simulink model "Md30StEnCtrl"  (R2018b)
settings: Solver=FixedStepDiscrete  StartTime=0.0  StopTime=10.0  FixedStep=0.01  RelTol=1e-3
undefined symbols (not defined in the file or in its folder): data, KeSMSuFirstRwStFwdBkwdPosDelta_Val, KeSMSw4SSecRwRtStLgrstOtwdInwdClosePos1_Val, KeSMSw4SSecRwRtStLgrstUpwdDnwdClosePos1_Val, KeSMSw4SSecRwRtStLgrstUpwdDnwdClosePos2_Val, KeSMSw4SSecRwRtStLgrstUpwdDnwdOpenPos1_Val, PassStBkReclnEn_Clear, PassStBkReclnEn_Set, PassStCshnFldEn_Clear, PassStCshnFldEn_Set, PassStFwdBkwdEn_Clear, PassStFwdBkwdEn_Set, SecRwRtStLgrstInwdOtwdEn_Clear, SecRwRtStLgrstInwdOtwdEn_Set, SecRwRtStLgrstUpwdDnwdEn_Clear, SecRwRtStLgrstUpwdDnwdEn_Set
libraries: simulink x3
settings Model: Creator=sn2xws  LastModifiedBy=sn55gm
settings Model: ModifiedHistory=|
  | 2024.6.27 V1.0.0 557模式流程V1.6
  | 2024.8.16 V3.0.0 增加firstTrig接口
  | 2024.8.19 V3.0.1前后位置判断时的减法加上括号保证运算顺序
  | 2024.11.6 V3.0.2模式流程V2.6 第一阶段增加收靠背动作
  | 2024.12.27 V3.0.3 BUG 965807 第一次靠背在位置判断应留余量
  | 25.07.15  V4.0.1 修改stage2前置条件
  | 25.7.31 V4.0.2 CR1100249
  | 25.8.11 V4.0.3 第一次完成后靠背到位置判断为alldone
  | 2025.09.03 V4.0.4 前后，折叠电机失败后退出
settings DataIOCC: SaveFormat=StructureWithTime
settings OptimizationCC: DefaultParameterBehavior=Inlined  EnhancedBackFolding=on  PassReuseOutputArgsAs=Individual arguments  ZeroExternalMemoryAtStartup=off  ZeroInternalMemoryAtStartup=off  OptimizeBlockOrder=speed  DifferentSizesBufferReuse=on  OptimizationCustomize=off
settings DebuggingCC: ParameterTunabilityLossMsg=error
settings SFSimCC: MATLABDynamicMemAlloc=off
settings RTWCC: SystemTargetFile=autosar.tlc  GenCodeOnly=on  TemplateMakefile=ert_default_tmf  Description=AUTOSAR  GenerateReport=on  IncludeHyperlinkInReport=on  LaunchReport=on  GenerateTraceInfo=on  GenerateTraceReport=on  GenerateTraceReportSl=on  GenerateTraceReportSf=on  GenerateTraceReportEml=on
settings CodeAppCC: ForceParamTrailComments=on  IgnoreCustomStorageClasses=off  OperatorAnnotations=on  SimulinkDataObjDesc=on  SFDataObjDesc=on  InsertBlockDesc=on
settings STFCustomTargetCC: TargetLangStandard=C99 (ISO)  MultiwordLength=256  ParMdlRefBuildCompliant=on  CompOptLevelCompliant=on  IncludeMdlTerminateFcn=off  CombineOutputUpdateFcns=on  SuppressErrorStatus=on  ERTCustomFileBanners=on  SupportNonFinite=off  SupportComplex=off  SupportContinuousTime=off  SupportNonInlinedSFcns=off  RemoveResetFunc=on  MATLABClassNameForMDSCustomization=Simulink.SoftwareTarget.ERTCustomization  AutosarCompliant=on  UseToolchainInfoCompliant=on  LookupTableObjectStructAxisOrder=2,1,3,4,...  LUTObjectStructOrderEvenSpacing=Size,Table,Breakpoints  SystemTargetFile=autosar.tlc
settings ERTTargetCC: TargetLangStandard=C99 (ISO)  ConcurrentExecutionCompliant=off  IncludeMdlTerminateFcn=off  SuppressErrorStatus=on  SupportNonFinite=off  SupportComplex=off  ModelStepFunctionPrototypeControlCompliant=off  CPPClassGenCompliant=off  AutosarCompliant=on  LookupTableObjectStructAxisOrder=2,1,3,4,...  LUTObjectStructOrderEvenSpacing=Size,Table,Breakpoints  InlinedParameterPlacement=NonHierarchical  ERTCustomFileTemplate=example_file_process.tlc  ERTFilePackagingFormat=Compact

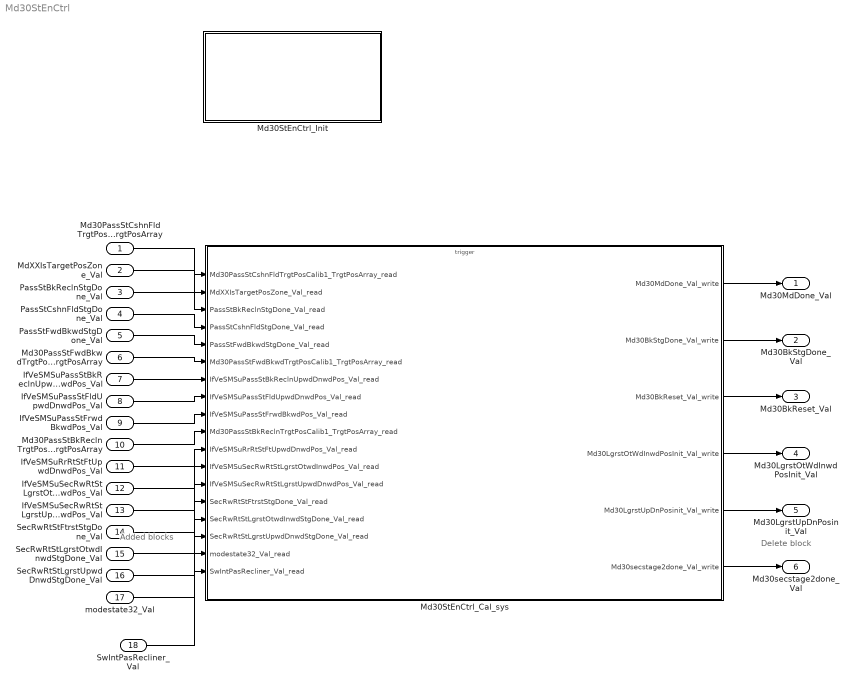
== system Md30StEnCtrl ==
  note: Delete block
  note: Added blocks
  Md30PassStCshnFldTrgtPosCalib1_TrgtPosArray : Inport  Description=|  OutDataTypeStr=uint16  PortDimensions=3
      | 0:Pos
      | 1:Max
      | 2:Min
  MdXXIsTargetPosZone_Val : Inport  Port=2  OutDataTypeStr=uint32  PortDimensions=1
  PassStBkReclnStgDone_Val : Inport  Port=3  OutDataTypeStr=boolean  PortDimensions=1
  PassStCshnFldStgDone_Val : Inport  Port=4  OutDataTypeStr=boolean  PortDimensions=1
  PassStFwdBkwdStgDone_Val : Inport  Port=5  OutDataTypeStr=boolean  PortDimensions=1
  Md30PassStFwdBkwdTrgtPosCalib1_TrgtPosArray : Inport  Description=|  Port=6  OutDataTypeStr=uint16  PortDimensions=3
      | 0:Pos
      | 1:Max
      | 2:Min
  IfVeSMSuPassStBkReclnUpwdDnwdPos_Val : Inport  Port=7  OutDataTypeStr=uint16  PortDimensions=1
  IfVeSMSuPassStFldUpwdDnwdPos_Val : Inport  Port=8  OutDataTypeStr=uint16  PortDimensions=1
  IfVeSMSuPassStFrwdBkwdPos_Val : Inport  Port=9  OutDataTypeStr=uint16  PortDimensions=1
  Md30PassStBkReclnTrgtPosCalib1_TrgtPosArray : Inport  Description=|  Port=10  OutDataTypeStr=uint16  PortDimensions=3
      | 0:Pos
      | 1:Max
      | 2:Min
  IfVeSMSuRrRtStFtUpwdDnwdPos_Val : Inport  Port=11  OutDataTypeStr=uint16  PortDimensions=1
  IfVeSMSuSecRwRtStLgrstOtwdInwdPos_Val : Inport  Port=12  OutDataTypeStr=uint16  PortDimensions=1
  IfVeSMSuSecRwRtStLgrstUpwdDnwdPos_Val : Inport  Port=13  OutDataTypeStr=uint16  PortDimensions=1
  SecRwRtStFtrstStgDone_Val : Inport  Port=14  OutDataTypeStr=boolean  PortDimensions=1
  SecRwRtStLgrstOtwdInwdStgDone_Val : Inport  Port=15  OutDataTypeStr=boolean  PortDimensions=1
  SecRwRtStLgrstUpwdDnwdStgDone_Val : Inport  Port=16  OutDataTypeStr=boolean  PortDimensions=1
  modestate32_Val : Inport  Port=17  OutDataTypeStr=uint32  PortDimensions=1
  SwIntPasRecliner_Val : Inport  Port=18  OutDataTypeStr=boolean  PortDimensions=1
  Md30StEnCtrl_Cal_sys : Subsystem
  Md30StEnCtrl_Init : Subsystem
  Md30MdDone_Val : Outport  OutDataTypeStr=uint8  PortDimensions=1
  Md30BkStgDone_Val : Outport  Port=2  OutDataTypeStr=boolean  PortDimensions=1
  Md30BkReset_Val : Outport  Port=3  OutDataTypeStr=boolean  PortDimensions=1
  Md30LgrstOtWdInwdPosInit_Val : Outport  Port=4  OutDataTypeStr=uint16  PortDimensions=1
  Md30LgrstUpDnPosinit_Val : Outport  Port=5  OutDataTypeStr=uint16  PortDimensions=1
  Md30secstage2done_Val : Outport  Port=6  OutDataTypeStr=boolean  PortDimensions=1
  wires:
  Md30PassStCshnFldTrgtPosCalib1_TrgtPosArray/1 -> Md30StEnCtrl_Cal_sys/1(Md30PassStCshnFldTrgtPosCalib1_TrgtPosArray_read)
  MdXXIsTargetPosZone_Val/1 -> Md30StEnCtrl_Cal_sys/2(MdXXIsTargetPosZone_Val_read)
  PassStBkReclnStgDone_Val/1 -> Md30StEnCtrl_Cal_sys/3(PassStBkReclnStgDone_Val_read)
  PassStCshnFldStgDone_Val/1 -> Md30StEnCtrl_Cal_sys/4(PassStCshnFldStgDone_Val_read)
  PassStFwdBkwdStgDone_Val/1 -> Md30StEnCtrl_Cal_sys/5(PassStFwdBkwdStgDone_Val_read)
  Md30StEnCtrl_Cal_sys/1(Md30MdDone_Val_write) -> Md30MdDone_Val/1
  Md30StEnCtrl_Cal_sys/2(Md30BkStgDone_Val_write) -> Md30BkStgDone_Val/1
  Md30PassStFwdBkwdTrgtPosCalib1_TrgtPosArray/1 -> Md30StEnCtrl_Cal_sys/6(Md30PassStFwdBkwdTrgtPosCalib1_TrgtPosArray_read)
  IfVeSMSuPassStBkReclnUpwdDnwdPos_Val/1 -> Md30StEnCtrl_Cal_sys/7(IfVeSMSuPassStBkReclnUpwdDnwdPos_Val_read)
  IfVeSMSuPassStFldUpwdDnwdPos_Val/1 -> Md30StEnCtrl_Cal_sys/8(IfVeSMSuPassStFldUpwdDnwdPos_Val_read)
  IfVeSMSuPassStFrwdBkwdPos_Val/1 -> Md30StEnCtrl_Cal_sys/9(IfVeSMSuPassStFrwdBkwdPos_Val_read)
  Md30PassStBkReclnTrgtPosCalib1_TrgtPosArray/1 -> Md30StEnCtrl_Cal_sys/10(Md30PassStBkReclnTrgtPosCalib1_TrgtPosArray_read)
  Md30StEnCtrl_Cal_sys/3(Md30BkReset_Val_write) -> Md30BkReset_Val/1
  IfVeSMSuRrRtStFtUpwdDnwdPos_Val/1 -> Md30StEnCtrl_Cal_sys/11(IfVeSMSuRrRtStFtUpwdDnwdPos_Val_read)
  IfVeSMSuSecRwRtStLgrstOtwdInwdPos_Val/1 -> Md30StEnCtrl_Cal_sys/12(IfVeSMSuSecRwRtStLgrstOtwdInwdPos_Val_read)
  IfVeSMSuSecRwRtStLgrstUpwdDnwdPos_Val/1 -> Md30StEnCtrl_Cal_sys/13(IfVeSMSuSecRwRtStLgrstUpwdDnwdPos_Val_read)
  SecRwRtStFtrstStgDone_Val/1 -> Md30StEnCtrl_Cal_sys/14(SecRwRtStFtrstStgDone_Val_read)
  SecRwRtStLgrstOtwdInwdStgDone_Val/1 -> Md30StEnCtrl_Cal_sys/15(SecRwRtStLgrstOtwdInwdStgDone_Val_read)
  SecRwRtStLgrstUpwdDnwdStgDone_Val/1 -> Md30StEnCtrl_Cal_sys/16(SecRwRtStLgrstUpwdDnwdStgDone_Val_read)
  modestate32_Val/1 -> Md30StEnCtrl_Cal_sys/17(modestate32_Val_read)
  Md30StEnCtrl_Cal_sys/4(Md30LgrstOtWdInwdPosInit_Val_write) -> Md30LgrstOtWdInwdPosInit_Val/1
  Md30StEnCtrl_Cal_sys/5(Md30LgrstUpDnPosinit_Val_write) -> Md30LgrstUpDnPosinit_Val/1
  Md30StEnCtrl_Cal_sys/6(Md30secstage2done_Val_write) -> Md30secstage2done_Val/1
  SwIntPasRecliner_Val/1 -> Md30StEnCtrl_Cal_sys/18(SwIntPasRecliner_Val_read)

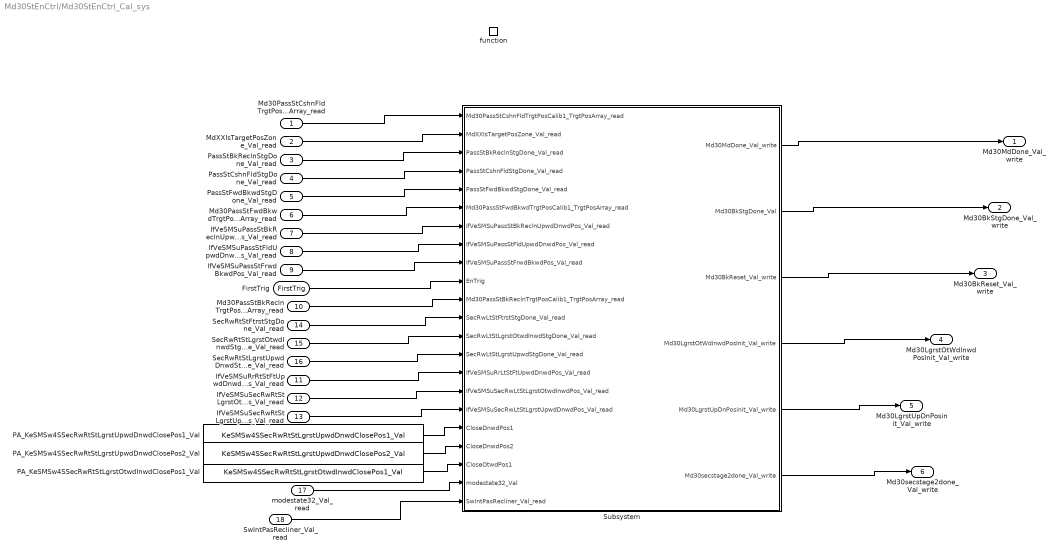
== system Md30StEnCtrl/Md30StEnCtrl_Cal_sys ==
  Md30PassStCshnFldTrgtPosCalib1_TrgtPosArray_read : Inport
  MdXXIsTargetPosZone_Val_read : Inport  Port=2
  PassStBkReclnStgDone_Val_read : Inport  Port=3
  PassStCshnFldStgDone_Val_read : Inport  Port=4
  PassStFwdBkwdStgDone_Val_read : Inport  Port=5
  Md30PassStFwdBkwdTrgtPosCalib1_TrgtPosArray_read : Inport  Port=6
  IfVeSMSuPassStBkReclnUpwdDnwdPos_Val_read : Inport  Port=7
  IfVeSMSuPassStFldUpwdDnwdPos_Val_read : Inport  Port=8
  IfVeSMSuPassStFrwdBkwdPos_Val_read : Inport  Port=9
  Md30PassStBkReclnTrgtPosCalib1_TrgtPosArray_read : Inport  Port=10
  IfVeSMSuRrRtStFtUpwdDnwdPos_Val_read : Inport  Port=11
  IfVeSMSuSecRwRtStLgrstOtwdInwdPos_Val_read : Inport  Port=12
  IfVeSMSuSecRwRtStLgrstUpwdDnwdPos_Val_read : Inport  Port=13
  SecRwRtStFtrstStgDone_Val_read : Inport  Port=14
  SecRwRtStLgrstOtwdInwdStgDone_Val_read : Inport  Port=15
  SecRwRtStLgrstUpwdDnwdStgDone_Val_read : Inport  Port=16
  modestate32_Val_read : Inport  Port=17
  SwIntPasRecliner_Val_read : Inport  Port=18
  function : TriggerPort  TriggerType=function-call  IsSimulinkFunction=on  FunctionName=Md30StEnCtrl_Cal  VariantControl=(inherit)
  PA_KeSMSw4SSecRwRtStLgrstOtwdInwdClosePos1_Val : Constant  Value=KeSMSw4SSecRwRtStLgrstOtwdInwdClosePos1_Val
  PA_KeSMSw4SSecRwRtStLgrstUpwdDnwdClosePos1_Val : Constant  Value=KeSMSw4SSecRwRtStLgrstUpwdDnwdClosePos1_Val
  PA_KeSMSw4SSecRwRtStLgrstUpwdDnwdClosePos2_Val : Constant  Value=KeSMSw4SSecRwRtStLgrstUpwdDnwdClosePos2_Val
  Subsystem : Subsystem
  FirstTrig : ArgIn  OutDataTypeStr=boolean  ArgumentName=FirstTrig
  Md30MdDone_Val_write : Outport
      settings: EnsureOutportIsVirtual=on
  Md30BkStgDone_Val_write : Outport  Port=2
      settings: EnsureOutportIsVirtual=on
  Md30BkReset_Val_write : Outport  Port=3
      settings: EnsureOutportIsVirtual=on
  Md30LgrstOtWdInwdPosInit_Val_write : Outport  Port=4
      settings: EnsureOutportIsVirtual=on
  Md30LgrstUpDnPosinit_Val_write : Outport  Port=5
      settings: EnsureOutportIsVirtual=on
  Md30secstage2done_Val_write : Outport  Port=6
      settings: EnsureOutportIsVirtual=on
  wires:
  Md30PassStCshnFldTrgtPosCalib1_TrgtPosArray_read/1 -> Subsystem/1(Md30PassStCshnFldTrgtPosCalib1_TrgtPosArray_read)
  MdXXIsTargetPosZone_Val_read/1 -> Subsystem/2(MdXXIsTargetPosZone_Val_read)
  PassStBkReclnStgDone_Val_read/1 -> Subsystem/3(PassStBkReclnStgDone_Val_read)
  PassStCshnFldStgDone_Val_read/1 -> Subsystem/4(PassStCshnFldStgDone_Val_read)
  PassStFwdBkwdStgDone_Val_read/1 -> Subsystem/5(PassStFwdBkwdStgDone_Val_read)
  Subsystem/1(Md30MdDone_Val_write) -> Md30MdDone_Val_write/1
  Subsystem/2(Md30BkStgDone_Val) -> Md30BkStgDone_Val_write/1
  Md30PassStFwdBkwdTrgtPosCalib1_TrgtPosArray_read/1 -> Subsystem/6(Md30PassStFwdBkwdTrgtPosCalib1_TrgtPosArray_read)
  IfVeSMSuPassStBkReclnUpwdDnwdPos_Val_read/1 -> Subsystem/7(IfVeSMSuPassStBkReclnUpwdDnwdPos_Val_read)
  IfVeSMSuPassStFldUpwdDnwdPos_Val_read/1 -> Subsystem/8(IfVeSMSuPassStFldUpwdDnwdPos_Val_read)
  IfVeSMSuPassStFrwdBkwdPos_Val_read/1 -> Subsystem/9(IfVeSMSuPassStFrwdBkwdPos_Val_read)
  Md30PassStBkReclnTrgtPosCalib1_TrgtPosArray_read/1 -> Subsystem/11(Md30PassStBkReclnTrgtPosCalib1_TrgtPosArray_read)
  FirstTrig/1 -> Subsystem/10(EnTrig)
  Subsystem/3(Md30BkReset_Val_write) -> Md30BkReset_Val_write/1
  IfVeSMSuRrRtStFtUpwdDnwdPos_Val_read/1 -> Subsystem/15(IfVeSMSuRrLtStFtUpwdDnwdPos_Val_read)
  IfVeSMSuSecRwRtStLgrstUpwdDnwdPos_Val_read/1 -> Subsystem/17(IfVeSMSuSecRwLtStLgrstUpwdDnwdPos_Val_read)
  SecRwRtStLgrstOtwdInwdStgDone_Val_read/1 -> Subsystem/13(SecRwLtStLgrstOtwdInwdStgDone_Val_read)
  SecRwRtStFtrstStgDone_Val_read/1 -> Subsystem/12(SecRwLtStFtrstStgDone_Val_read)
  SecRwRtStLgrstUpwdDnwdStgDone_Val_read/1 -> Subsystem/14(SecRwLtStLgrstUpwdStgDone_Val_read)
  IfVeSMSuSecRwRtStLgrstOtwdInwdPos_Val_read/1 -> Subsystem/16(IfVeSMSuSecRwLtStLgrstOtwdInwdPos_Val_read)
  PA_KeSMSw4SSecRwRtStLgrstUpwdDnwdClosePos1_Val/1 -> Subsystem/18(CloseDnwdPos1)
  PA_KeSMSw4SSecRwRtStLgrstOtwdInwdClosePos1_Val/1 -> Subsystem/20(CloseOtwdPos1)
  PA_KeSMSw4SSecRwRtStLgrstUpwdDnwdClosePos2_Val/1 -> Subsystem/19(CloseDnwdPos2)
  modestate32_Val_read/1 -> Subsystem/21(modestate32_Val)
  Subsystem/4(Md30LgrstOtWdInwdPosInit_Val_write) -> Md30LgrstOtWdInwdPosInit_Val_write/1
  Subsystem/5(Md30LgrstUpDnPosinit_Val_write) -> Md30LgrstUpDnPosinit_Val_write/1
  Subsystem/6(Md30secstage2done_Val_write) -> Md30secstage2done_Val_write/1
  SwIntPasRecliner_Val_read/1 -> Subsystem/22(SwIntPasRecliner_Val_read)

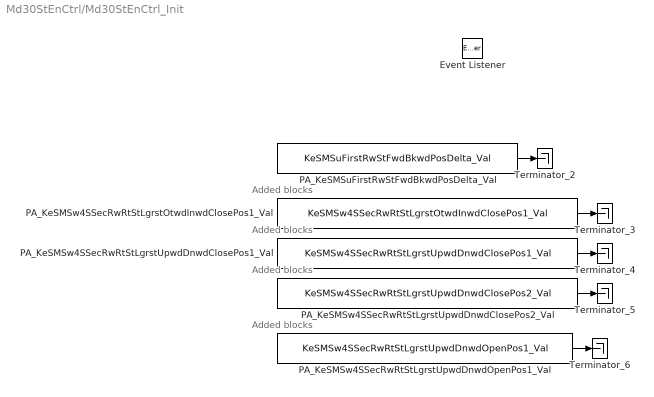
== system Md30StEnCtrl/Md30StEnCtrl_Init ==
  note: Added blocks
  note: Added blocks
  note: Added blocks
  note: Added blocks
  Event Listener : EventListener  EventName=reset
  PA_KeSMSuFirstRwStFwdBkwdPosDelta_Val : Constant  Value=KeSMSuFirstRwStFwdBkwdPosDelta_Val
  PA_KeSMSw4SSecRwRtStLgrstOtwdInwdClosePos1_Val : Constant  Value=KeSMSw4SSecRwRtStLgrstOtwdInwdClosePos1_Val
  PA_KeSMSw4SSecRwRtStLgrstUpwdDnwdClosePos1_Val : Constant  Value=KeSMSw4SSecRwRtStLgrstUpwdDnwdClosePos1_Val
  PA_KeSMSw4SSecRwRtStLgrstUpwdDnwdClosePos2_Val : Constant  Value=KeSMSw4SSecRwRtStLgrstUpwdDnwdClosePos2_Val
  PA_KeSMSw4SSecRwRtStLgrstUpwdDnwdOpenPos1_Val : Constant  Value=KeSMSw4SSecRwRtStLgrstUpwdDnwdOpenPos1_Val
  Terminator_{2..6} (5 alike) : Terminator
  wires:
  PA_KeSMSuFirstRwStFwdBkwdPosDelta_Val/1 -> Terminator_2/1
  PA_KeSMSw4SSecRwRtStLgrstOtwdInwdClosePos1_Val/1 -> Terminator_3/1
  PA_KeSMSw4SSecRwRtStLgrstUpwdDnwdClosePos1_Val/1 -> Terminator_4/1
  PA_KeSMSw4SSecRwRtStLgrstUpwdDnwdClosePos2_Val/1 -> Terminator_5/1
  PA_KeSMSw4SSecRwRtStLgrstUpwdDnwdOpenPos1_Val/1 -> Terminator_6/1

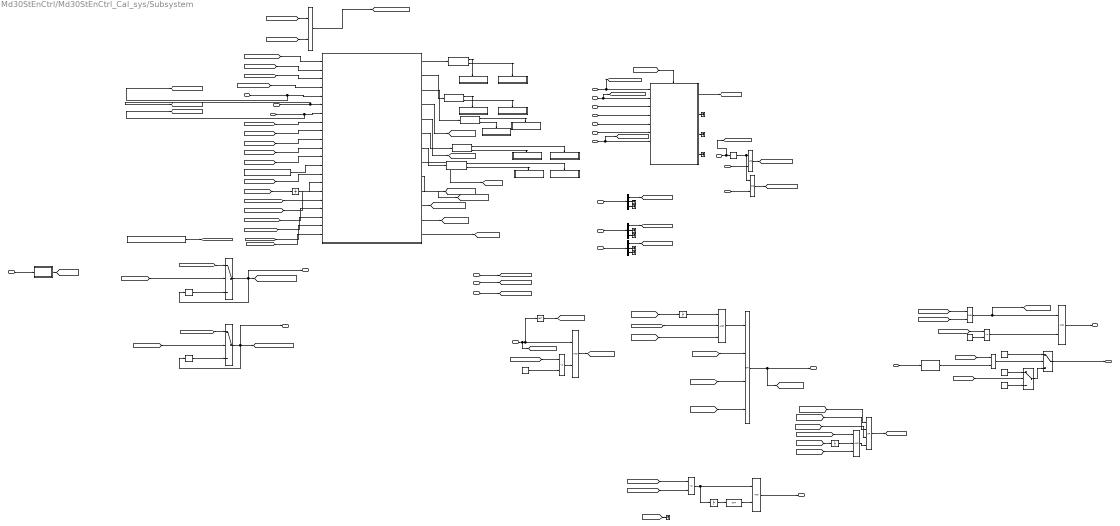
== system Md30StEnCtrl/Md30StEnCtrl_Cal_sys/Subsystem ==
  Md30PassStCshnFldTrgtPosCalib1_TrgtPosArray_read : Inport
  MdXXIsTargetPosZone_Val_read : Inport  Port=2
  PassStBkReclnStgDone_Val_read : Inport  Port=3
  PassStCshnFldStgDone_Val_read : Inport  Port=4
  PassStFwdBkwdStgDone_Val_read : Inport  Port=5
  Md30PassStFwdBkwdTrgtPosCalib1_TrgtPosArray_read : Inport  Port=6
  IfVeSMSuPassStBkReclnUpwdDnwdPos_Val_read : Inport  Port=7
  IfVeSMSuPassStFldUpwdDnwdPos_Val_read : Inport  Port=8
  IfVeSMSuPassStFrwdBkwdPos_Val_read : Inport  Port=9
  EnTrig : Inport  Port=10
  Md30PassStBkReclnTrgtPosCalib1_TrgtPosArray_read : Inport  Port=11
  SecRwLtStFtrstStgDone_Val_read : Inport  Port=12
  SecRwLtStLgrstOtwdInwdStgDone_Val_read : Inport  Port=13
  SecRwLtStLgrstUpwdStgDone_Val_read : Inport  Port=14
  IfVeSMSuRrLtStFtUpwdDnwdPos_Val_read : Inport  Port=15
  IfVeSMSuSecRwLtStLgrstOtwdInwdPos_Val_read : Inport  Port=16
  IfVeSMSuSecRwLtStLgrstUpwdDnwdPos_Val_read : Inport  Port=17
  CloseDnwdPos1 : Inport  Port=18
  CloseDnwdPos2 : Inport  Port=19
  CloseOtwdPos1 : Inport  Port=20
  modestate32_Val : Inport  Port=21
  SwIntPasRecliner_Val_read : Inport  Port=22
  32BitSelector : Subsystem  mask(32 Bit Selector){BitNum=29}
      mask prompts: BitNum "Select Bit Number"
      mask help: Allows selection of a particular bit (0-31) out of a packed word up to 32 bits long. Output will be true if the bit number selected via the mask parameter is equal to one.
      mask TypeOptions BitNum: 0 | 1 | 2 | 3 | 4 | 5 | 6 | 7 | 8 | 9 | 10 | 11 | 12 | 13 | 14 | 15 | 16 | 17 | 18 | 19 | 20 | 21 | 22 | 23 | 24 | 25 | 26 | 27 | 28 | 29 | 30 | 31
      mask Display:
      | text(0.5, 0.8,'BIT','horizontalAlignment','center')
      | text(0.5, 0.5,'SELECTOR','horizontalAlignment','center')
      | text(0.5, 0.2,['-- Bit ',char(get_param(gcb,'BitNum')),' --'],'horizontalAlignment','center')
  32BitSelector1 : Subsystem  mask(32 Bit Selector){BitNum=29}
      mask prompts: BitNum "Select Bit Number"
      mask help: Allows selection of a particular bit (0-31) out of a packed word up to 32 bits long. Output will be true if the bit number selected via the mask parameter is equal to one.
      mask TypeOptions BitNum: 0 | 1 | 2 | 3 | 4 | 5 | 6 | 7 | 8 | 9 | 10 | 11 | 12 | 13 | 14 | 15 | 16 | 17 | 18 | 19 | 20 | 21 | 22 | 23 | 24 | 25 | 26 | 27 | 28 | 29 | 30 | 31
      mask Display:
      | text(0.5, 0.8,'BIT','horizontalAlignment','center')
      | text(0.5, 0.5,'SELECTOR','horizontalAlignment','center')
      | text(0.5, 0.2,['-- Bit ',char(get_param(gcb,'BitNum')),' --'],'horizontalAlignment','center')
  Chart : Stateflow chart  TreatAsAtomicUnit=on
  Compare To Constant : simulink/Logic and Bit Operations/Compare To Constant  relop===  const=1  OutDataTypeStr=boolean
  Constant : Constant  Value=40  OutDataTypeStr=uint16
  Constant1 : Constant  OutDataTypeStr=uint8
  Constant2 : Constant  Value=2  OutDataTypeStr=uint8
  Constant3 : Constant  Value=0  OutDataTypeStr=uint8
  Constant4 : Constant  Value=120  OutDataTypeStr=uint16
  Delay1 : Delay  DelayLength=1
  Delay3 : Delay  DelayLength=1
  Demux : Demux  Outputs=3
  Demux1 : Demux  Outputs=3
  Demux2 : Demux  Outputs=3
  If Action Subsystem1 : Subsystem  TreatAsAtomicUnit=on
  If Action Subsystem11 : Subsystem  TreatAsAtomicUnit=on
  If Action Subsystem14 : Subsystem  TreatAsAtomicUnit=on
  If Action Subsystem2 : Subsystem  TreatAsAtomicUnit=on
  If Action Subsystem3 : Subsystem  TreatAsAtomicUnit=on
  If Action Subsystem4 : Subsystem  TreatAsAtomicUnit=on
  If Action Subsystem5 : Subsystem  TreatAsAtomicUnit=on
  If Action Subsystem6 : Subsystem  TreatAsAtomicUnit=on
  If Action Subsystem7 : Subsystem  TreatAsAtomicUnit=on
  If Action Subsystem8 : Subsystem  TreatAsAtomicUnit=on
  If{1..4,8} (5 alike) : If  IfExpression=u1
  Logical Operator{,3,5,9,13,24} (6 alike) : Logic  AllPortsSameDT=off  OutDataTypeStr=boolean
  Logical Operator1 : Logic  Inputs=3  AllPortsSameDT=off  OutDataTypeStr=boolean
  Logical Operator10 : Logic  Operator=OR  AllPortsSameDT=off  OutDataTypeStr=boolean
  Logical Operator2 : Logic  Operator=OR  Inputs=4  AllPortsSameDT=off  OutDataTypeStr=boolean
  Logical Operator22 : Logic  Inputs=3  AllPortsSameDT=off  OutDataTypeStr=boolean
  Logical Operator4 : Logic  Operator=NOT  AllPortsSameDT=off  OutDataTypeStr=boolean
  Logical Operator6 : Logic  Operator=NOT  AllPortsSameDT=off  OutDataTypeStr=boolean
  Logical Operator7 : Logic  Operator=OR  Inputs=4  AllPortsSameDT=off  OutDataTypeStr=boolean
  Logical Operator8 : Logic  Operator=OR  AllPortsSameDT=off  OutDataTypeStr=boolean
  PA_KeSMSuFirstRwStFwdBkwdPosDelta_Val : Constant  Value=KeSMSuFirstRwStFwdBkwdPosDelta_Val
  PA_KeSMSw4SSecRwRtStLgrstUpwdDnwdClosePos1_Val : Constant  Value=KeSMSw4SSecRwRtStLgrstUpwdDnwdOpenPos1_Val
  Relational Operator : RelationalOperator  Operator=<=  OutDataTypeStr=boolean  RndMeth=Simplest
  Relational Operator1 : RelationalOperator  Operator=<=  OutDataTypeStr=boolean  RndMeth=Simplest
  Relational Operator2 : RelationalOperator  Operator=<=  OutDataTypeStr=boolean  RndMeth=Simplest
  Subsystem : Subsystem
  Switch{,1..3} (4 alike) : Switch  Criteria=u2 > Threshold
  Terminator_{1..2,4..5,7..12} (10 alike) : Terminator
  Unit Delay{,1..3} (4 alike) : UnitDelay  SampleTime=-1
  Md30MdDone_Val_write : Outport
      settings: EnsureOutportIsVirtual=on
  Md30BkStgDone_Val : Outport  Port=2
      settings: EnsureOutportIsVirtual=on
  Md30BkReset_Val_write : Outport  Port=3
      settings: EnsureOutportIsVirtual=on
  Md30LgrstOtWdInwdPosInit_Val_write : Outport  Port=4
  Md30LgrstUpDnPosinit_Val_write : Outport  Port=5
  Md30secstage2done_Val_write : Outport  Port=6
  wires:
  Switch/1 -> Md30MdDone_Val_write/1
  PassStBkReclnStgDone_Val_read/1 -> [PassStBkReclnStgDone], Chart/5(PassStBkReclnStgDone)
  PassStCshnFldStgDone_Val_read/1 -> Chart/6(PassStCshnFldStgDone), [PassStCshnFldStgDone]
  PassStFwdBkwdStgDone_Val_read/1 -> Chart/7(PassStFwdBkwdStgDone), [PassStFwdBkwdStgDone]
  [AllDone] -> Logical Operator9/1
  Constant1/1 -> Switch/1
  Constant2/1 -> Switch1/1
  Switch1/1 -> Switch/3
  Constant3/1 -> Switch1/3
  Logical Operator9/1 -> Switch/2
  MdXXIsTargetPosZone_Val_read/1 -> 32BitSelector/1(x)
  [AllDone] -> Switch1/2
  Md30PassStFwdBkwdTrgtPosCalib1_TrgtPosArray_read/1 -> Demux/1
  Demux/1 -> [PassStFwdBkwdTrgtPos1]
  Demux1/1 -> [PassStCshnFldTrgtPos1]
  Md30PassStCshnFldTrgtPosCalib1_TrgtPosArray_read/1 -> Demux1/1
  [PassStFwdBkwdTrgtPos1] -> Chart/8(PassStFwdBkwdTrgtPos1)
  [PassStCshnFldTrgtPos1] -> Chart/9(PassStCshnFldTrgtPos1)
  IfVeSMSuPassStFrwdBkwdPos_Val_read/1 -> [PassStFwdBkwdPos]
  IfVeSMSuPassStFldUpwdDnwdPos_Val_read/1 -> [PassStFldUpwdDnwdPos]
  [PassStFldUpwdDnwdPos] -> Chart/10(PassStFldUpwdDnwdPos)
  [PassStFwdBkwdPos] -> Chart/11(PassStFwdBkwdPos)
  IfVeSMSuPassStBkReclnUpwdDnwdPos_Val_read/1 -> [PassStBkReclnUpwdDnwdPos]
  [PassStBkReclnUpwdDnwdPos] -> Chart/12(PassStBkReclnUpwdDnwdPos)
  Logical Operator/1 -> Logical Operator13/1, [BkStgDone]
  [PassStCshnFldStgDone] -> Logical Operator/2
  [BkStgDone] -> Unit Delay/1
  Unit Delay/1 -> Logical Operator1/1
  [PassStFwdBkwdStgDone] -> Logical Operator1/2
  Chart/1(PassStBkReclnEn) -> If8/1
  If8/1 -> If Action Subsystem14/Action
  If8/2 -> If Action Subsystem11/Action
  If1/2 -> If Action Subsystem1/Action
  If1/1 -> If Action Subsystem2/Action
  Chart/2(PassStCshnFldEn) -> If1/1
  If2/1 -> If Action Subsystem4/Action
  If2/2 -> If Action Subsystem3/Action
  Chart/3(PassStFwdBkwdEn) -> If2/1
  Demux/2 -> Terminator_4/1
  Demux/3 -> Terminator_5/1
  Demux1/2 -> Terminator_7/1
  Demux1/3 -> Terminator_8/1
  PA_KeSMSuFirstRwStFwdBkwdPosDelta_Val/1 -> Chart/13(KeSMSuFirstRwStFwdBkwdPosDelta)
  Chart/4(FwdBkwdFailflg) -> [FwdBkwdFailflg]
  Chart/5(CshnFldFailflg) -> [CshnFldFailflg]
  Logical Operator1/1 -> Logical Operator2/1
  [FwdBkwdFailflg] -> Logical Operator2/2
  [CshnFldFailflg] -> Logical Operator2/3
  [PassStBkReclnUpwdDnwdPos] -> Relational Operator/1
  Constant/1 -> Relational Operator/2
  [FirstBkDone] -> Logical Operator2/4
  Relational Operator/1 -> Logical Operator3/2
  Logical Operator3/1 -> [FirstBkDone]
  32BitSelector/1(y) -> Logical Operator9/2
  [PassStBkReclnStgDone] -> Logical Operator/1
  Demux2/3 -> Terminator_2/1
  Demux2/2 -> Terminator_1/1
  Demux2/1 -> [Md30PassStBkReclnTrgtPos1]
  Md30PassStBkReclnTrgtPosCalib1_TrgtPosArray_read/1 -> Demux2/1
  [Md30PassStBkReclnTrgtPos1] -> Chart/14(Md30PassStBkReclnTrgtPos1)
  [PassStFldUpwdDnwdPos] -> Relational Operator1/1
  [PassStCshnFldTrgtPos1] -> Relational Operator1/2
  Relational Operator1/1 -> Logical Operator5/1, Unit Delay1/1
  Unit Delay1/1 -> Logical Operator4/1
  Logical Operator4/1 -> Logical Operator5/2
  Logical Operator5/1 -> Md30BkReset_Val_write/1
  [NotFirstTime] -> Logical Operator1/3
  Logical Operator6/1 -> [NotFirstTime]
  SecRwLtStLgrstOtwdInwdStgDone_Val_read/1 -> Subsystem/7(In7), [SecRwLtStLgrstOtwdInwdStgDone]
  IfVeSMSuSecRwLtStLgrstUpwdDnwdPos_Val_read/1 -> [LgrstUpDnPos], Subsystem/1(In1)
  IfVeSMSuSecRwLtStLgrstOtwdInwdPos_Val_read/1 -> Subsystem/2(In2), [LgrstOtWdInwdPos]
  IfVeSMSuRrLtStFtUpwdDnwdPos_Val_read/1 -> Subsystem/3(In3)
  CloseDnwdPos1/1 -> Subsystem/4(In4)
  CloseDnwdPos2/1 -> Subsystem/5(In5)
  CloseOtwdPos1/1 -> Subsystem/6(In6)
  Subsystem/1(Out1) -> [failflg]
  Chart/13(TrigLgrstcls()) -> [TrigLgrstcls]
  [TrigLgrstcls] -> Subsystem/Trigger
  [stage2Done] -> Unit Delay3/1
  Relational Operator2/1 -> Logical Operator13/2
  [PassStBkReclnUpwdDnwdPos] -> Relational Operator2/1
  Constant4/1 -> Relational Operator2/2
  Logical Operator13/1 -> Md30BkStgDone_Val/1
  [SecRwLtStFtrstStgDone] -> Chart/4(SecRwLtStFtrstStgDone)
  [SecRwLtStLgrstUpwdStgDone] -> Chart/2(SecRwLtStLgrstUpwdStgDone)
  [SecRwLtStLgrstOtwdInwdStgDone] -> Chart/3(SecRwLtStLgrstOtwdInwdStgDone)
  modestate32_Val/1 -> 32BitSelector1/1(x)
  32BitSelector1/1(y) -> [Mode30]
  [EnTrig] -> Switch2/2
  [LgrstOtWdInwdPos] -> Switch2/1
  Delay1/1 -> Switch2/3
  Delay3/1 -> Switch3/3
  [LgrstUpDnPos] -> Switch3/1
  Switch2/1 -> Md30LgrstOtWdInwdPosInit_Val_write/1, Delay1/1, [LgrstOtWdInwdPosInit]
  [LgrstOtWdInwdPosInit] -> Chart/16(LgrstOtWdInwdPosInit)
  [LgrstUpDnPosinit] -> Chart/17(LgrstUpDnPosinit)
  [LgrstOtWdInwdPos] -> Chart/18(LgrstOtWdInwdPos)
  [LgrstUpDnPos] -> Chart/19(LgrstUpDnPos)
  Switch3/1 -> Delay3/1, Md30LgrstUpDnPosinit_Val_write/1, [LgrstUpDnPosinit]
  [LgrstUpwdDnwdOpenPos1] -> Chart/20(LgrstUpwdDnwdOpenPos1)
  Chart/6(SecRwLtStLgrstUpwdEn) -> If3/1
  Chart/8(LgrstUpwdfailflg) -> [LgrstUpwdfailflg]
  Chart/9(stage2LgrstUpwdStgDone) -> [stage2LgrstUpwdStgDone]
  Chart/10(stage2LgrstOtwdInwdStgDone) -> [stage2LgrstOtwdInwdStgDone]
  Logical Operator2/1 -> [stage2Done], Md30secstage2done_Val_write/1
  [stage2Done] -> Unit Delay2/1
  [LgrstUpwdfailflg] -> Terminator_9/1
  PA_KeSMSw4SSecRwRtStLgrstUpwdDnwdClosePos1_Val/1 -> [LgrstUpwdDnwdOpenPos1]
  [SecRwLtStLgrstOtwdInwdStgDone] -> Logical Operator24/2
  [SecRwLtStLgrstUpwdStgDone] -> Logical Operator24/1
  [stage1Done] -> Chart/1(stage1Done)
  If3/1 -> If Action Subsystem5/Action
  If4/2 -> If Action Subsystem8/Action
  If4/1 -> If Action Subsystem7/Action
  Chart/7(SecRwLtStLgrstOtwdInwdEn) -> If4/1
  Subsystem/2(Out2) -> Terminator_10/1
  Subsystem/3(Out3) -> Terminator_11/1
  Subsystem/4(Out4) -> Terminator_12/1
  Unit Delay3/1 -> Chart/15(stage2Done)
  EnTrig/1 -> [EnTrig], Logical Operator6/1, Logical Operator3/1
  [EnTrig] -> Switch3/2
  If3/2 -> If Action Subsystem6/Action
  [stage1Done] -> Logical Operator22/1
  Unit Delay2/1 -> Logical Operator22/2
  [NotFirstTime] -> Logical Operator22/3
  Chart/11(LgrstUpDnPosfail) -> [LgrstUpDnPosfail]
  Chart/12(LgrstOtWdInwdPosfail) -> [LgrstOtWdInwdPosfail]
  Logical Operator24/1 -> [stage1Done]
  Logical Operator22/1 -> Logical Operator7/4
  [FirstBkDone] -> Logical Operator7/3
  Logical Operator7/1 -> [AllDone]
  [FwdBkwdFailflg] -> Logical Operator7/2
  [CshnFldFailflg] -> Logical Operator7/1
  Compare To Constant/1 -> Logical Operator10/1, Logical Operator8/1
  SecRwLtStLgrstUpwdStgDone_Val_read/1 -> Logical Operator8/2
  Logical Operator8/1 -> [SecRwLtStLgrstUpwdStgDone]
  SecRwLtStFtrstStgDone_Val_read/1 -> Logical Operator10/2
  Logical Operator10/1 -> [SecRwLtStFtrstStgDone]
  SwIntPasRecliner_Val_read/1 -> [SwIntPasRecliner], Compare To Constant/1
  [SwIntPasRecliner] -> Chart/21(SwIntPasRecliner)

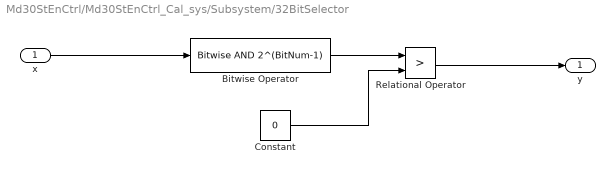
== system Md30StEnCtrl/Md30StEnCtrl_Cal_sys/Subsystem/32BitSelector ==
  x : Inport
  Bitwise Operator : simulink/Logic and Bit Operations/Bitwise Operator  logicop=AND  UseBitMask=on  BitMask=2^(BitNum-1)  BitMaskRealWorld=Stored Integer
  Constant : Constant  Value=0  OutDataTypeStr=uint32
  Relational Operator : RelationalOperator  Operator=>  OutDataTypeStr=boolean  RndMeth=Simplest
  y : Outport
  wires:
  Relational Operator/1 -> y/1
  Constant/1 -> Relational Operator/2
  x/1 -> Bitwise Operator/1
  Bitwise Operator/1 -> Relational Operator/1

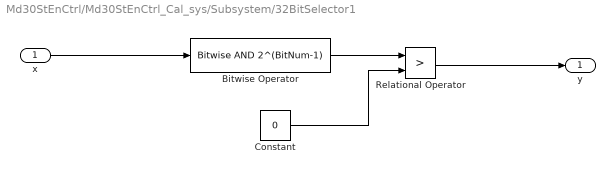
== system Md30StEnCtrl/Md30StEnCtrl_Cal_sys/Subsystem/32BitSelector1 ==
  x : Inport
  Bitwise Operator : simulink/Logic and Bit Operations/Bitwise Operator  logicop=AND  UseBitMask=on  BitMask=2^(BitNum-1)  BitMaskRealWorld=Stored Integer
  Constant : Constant  Value=0  OutDataTypeStr=uint32
  Relational Operator : RelationalOperator  Operator=>  OutDataTypeStr=boolean  RndMeth=Simplest
  y : Outport
  wires:
  Relational Operator/1 -> y/1
  Constant/1 -> Relational Operator/2
  x/1 -> Bitwise Operator/1
  Bitwise Operator/1 -> Relational Operator/1

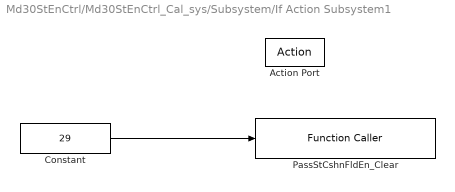
== system Md30StEnCtrl/Md30StEnCtrl_Cal_sys/Subsystem/If Action Subsystem1 ==
  Action Port : ActionPort  ActionType=else
  Constant : Constant  Value=29  OutDataTypeStr=uint8
  PassStCshnFldEn_Clear : FunctionCaller  FunctionPrototype=PassStCshnFldEn_Clear(data)  InputArgumentSpecifications=uint8(1)
  wires:
  Constant/1 -> PassStCshnFldEn_Clear/1

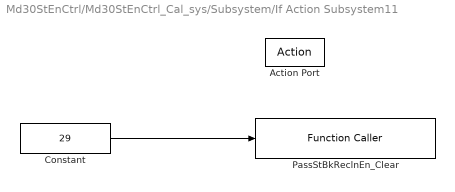
== system Md30StEnCtrl/Md30StEnCtrl_Cal_sys/Subsystem/If Action Subsystem11 ==
  Action Port : ActionPort  ActionType=else
  Constant : Constant  Value=29  OutDataTypeStr=uint8
  PassStBkReclnEn_Clear : FunctionCaller  FunctionPrototype=PassStBkReclnEn_Clear(data)  InputArgumentSpecifications=uint8(1)
  wires:
  Constant/1 -> PassStBkReclnEn_Clear/1

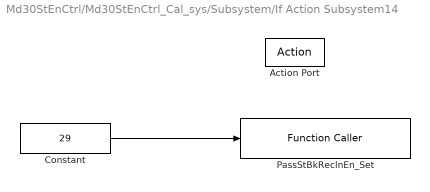
== system Md30StEnCtrl/Md30StEnCtrl_Cal_sys/Subsystem/If Action Subsystem14 ==
  Action Port : ActionPort  ActionType=then
  Constant : Constant  Value=29  OutDataTypeStr=uint8
  PassStBkReclnEn_Set : FunctionCaller  FunctionPrototype=PassStBkReclnEn_Set(data)  InputArgumentSpecifications=uint8(1)
  wires:
  Constant/1 -> PassStBkReclnEn_Set/1

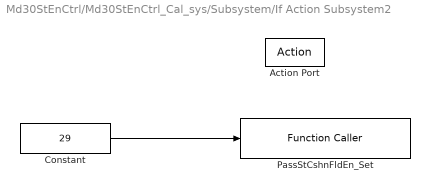
== system Md30StEnCtrl/Md30StEnCtrl_Cal_sys/Subsystem/If Action Subsystem2 ==
  Action Port : ActionPort  ActionType=then
  Constant : Constant  Value=29  OutDataTypeStr=uint8
  PassStCshnFldEn_Set : FunctionCaller  FunctionPrototype=PassStCshnFldEn_Set(data)  InputArgumentSpecifications=uint8(1)
  wires:
  Constant/1 -> PassStCshnFldEn_Set/1

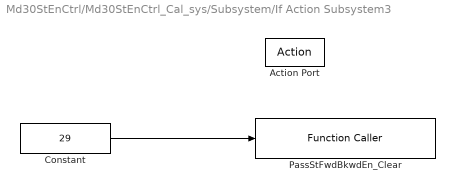
== system Md30StEnCtrl/Md30StEnCtrl_Cal_sys/Subsystem/If Action Subsystem3 ==
  Action Port : ActionPort  ActionType=else
  Constant : Constant  Value=29  OutDataTypeStr=uint8
  PassStFwdBkwdEn_Clear : FunctionCaller  FunctionPrototype=PassStFwdBkwdEn_Clear(data)  InputArgumentSpecifications=uint8(1)
  wires:
  Constant/1 -> PassStFwdBkwdEn_Clear/1

== system Md30StEnCtrl/Md30StEnCtrl_Cal_sys/Subsystem/If Action Subsystem4 ==
  Action Port : ActionPort  ActionType=then
  Constant : Constant  Value=29  OutDataTypeStr=uint8
  PassStFwdBkwdEn_Set : FunctionCaller  FunctionPrototype=PassStFwdBkwdEn_Set(data)  InputArgumentSpecifications=uint8(1)
  wires:
  Constant/1 -> PassStFwdBkwdEn_Set/1

== system Md30StEnCtrl/Md30StEnCtrl_Cal_sys/Subsystem/If Action Subsystem5 ==
  Action Port : ActionPort  ActionType=then
  Constant : Constant  Value=29  OutDataTypeStr=uint8
  SecRwRtStLgrstUpwdDnwdEn_Set : FunctionCaller  FunctionPrototype=SecRwRtStLgrstUpwdDnwdEn_Set(data)  InputArgumentSpecifications=uint8(1)
  wires:
  Constant/1 -> SecRwRtStLgrstUpwdDnwdEn_Set/1

== system Md30StEnCtrl/Md30StEnCtrl_Cal_sys/Subsystem/If Action Subsystem6 ==
  Action Port : ActionPort  ActionType=else
  Constant : Constant  Value=29  OutDataTypeStr=uint8
  SecRwRtStLgrstUpwdDnwdEn_Clear : FunctionCaller  FunctionPrototype=SecRwRtStLgrstUpwdDnwdEn_Clear(data)  InputArgumentSpecifications=uint8(1)
  wires:
  Constant/1 -> SecRwRtStLgrstUpwdDnwdEn_Clear/1

== system Md30StEnCtrl/Md30StEnCtrl_Cal_sys/Subsystem/If Action Subsystem7 ==
  Action Port : ActionPort  ActionType=then
  Constant : Constant  Value=29  OutDataTypeStr=uint8
  SecRwRtStLgrstInwdOtwdEn_Set : FunctionCaller  FunctionPrototype=SecRwRtStLgrstInwdOtwdEn_Set(data)  InputArgumentSpecifications=uint8(1)
  wires:
  Constant/1 -> SecRwRtStLgrstInwdOtwdEn_Set/1

== system Md30StEnCtrl/Md30StEnCtrl_Cal_sys/Subsystem/If Action Subsystem8 ==
  Action Port : ActionPort  ActionType=else
  Constant : Constant  Value=29  OutDataTypeStr=uint8
  SecRwRtStLgrstInwdOtwdEn_Clear : FunctionCaller  FunctionPrototype=SecRwRtStLgrstInwdOtwdEn_Clear(data)  InputArgumentSpecifications=uint8(1)
  wires:
  Constant/1 -> SecRwRtStLgrstInwdOtwdEn_Clear/1

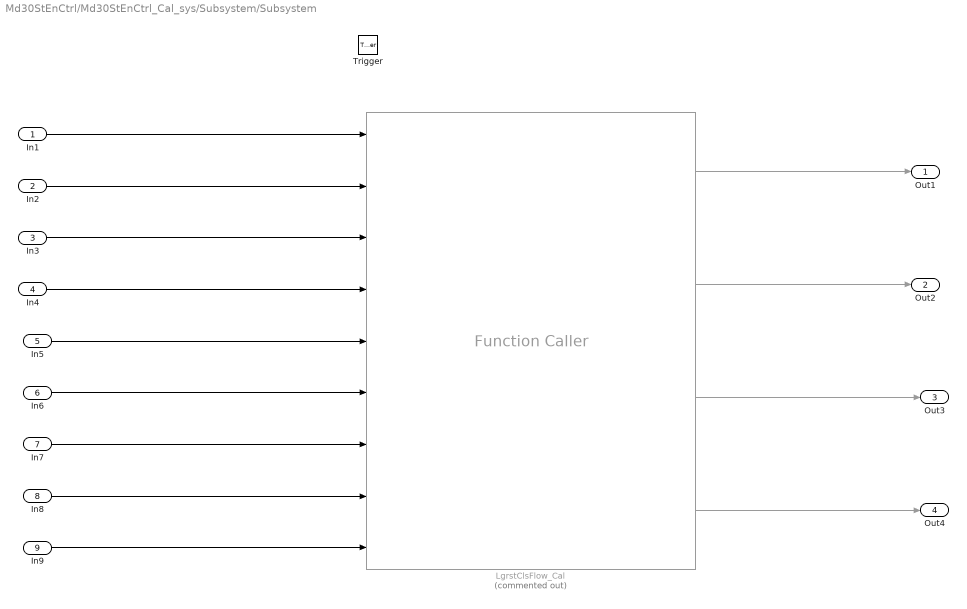
== system Md30StEnCtrl/Md30StEnCtrl_Cal_sys/Subsystem/Subsystem ==
  In1 : Inport
  In2 : Inport  Port=2
  In3 : Inport  Port=3
  In4 : Inport  Port=4
  In5 : Inport  Port=5
  In6 : Inport  Port=6
  In7 : Inport  Port=7
  In8 : Inport  Port=8
  In9 : Inport  Port=9
  Trigger : TriggerPort  TriggerType=function-call  VariantControl=Variant  PortDimensions=1
  LgrstClsFlow_Cal : FunctionCaller  Commented=on  FunctionPrototype=[Failflg,LgrstInwdOtwdEn,LgrstUpwdDnwdEn,FtrstEn] = LgrstClsFlow_Cal(LgrstUpwdDnwdPos,LgrstOtwdInwdPos,FtUpwdDnwdPos,CloseDnwdPos1,CloseDnwdPos2,CloseOtwdPos1,LgrstInwdStgDone,LgrstUpwdStgDone,FtrstStgDone)  InputArgumentSpecifications=uint16(1), uint16(1), uint16(1), uint16(1), uint16(1), uint16(1), boolean(true), boolean(true), boolean(true)  OutputArgumentSpecifications=boolean(true), boolean(true), boolean(true), boolean(true)
  Out1 : Outport
  Out2 : Outport  Port=2
  Out3 : Outport  Port=3
  Out4 : Outport  Port=4
  wires:
  In8/1 -> LgrstClsFlow_Cal/8
  In1/1 -> LgrstClsFlow_Cal/1
  In7/1 -> LgrstClsFlow_Cal/7
  LgrstClsFlow_Cal/3 -> Out3/1
  In2/1 -> LgrstClsFlow_Cal/2
  LgrstClsFlow_Cal/4 -> Out4/1
  In9/1 -> LgrstClsFlow_Cal/9
  LgrstClsFlow_Cal/2 -> Out2/1
  In5/1 -> LgrstClsFlow_Cal/5
  In4/1 -> LgrstClsFlow_Cal/4
  LgrstClsFlow_Cal/1 -> Out1/1
  In6/1 -> LgrstClsFlow_Cal/6
  In3/1 -> LgrstClsFlow_Cal/3

== stateflow chart Md30StEnCtrl/Md30StEnCtrl_Cal_sys/Subsystem/Chart ==
  (default) -> (junction 92) : {
      | PassStFwdBkwdEn = 0;
      | PassStBkReclnEn = 0;
      | PassStCshnFldEn = 0;
      | FwdBkwdFailflg = 0;
      | CshnFldFailflg = 0;
      | SecRwLtStLgrstUpwdEn = 0;
      | SecRwLtStLgrstOtwdInwdEn = 0;
      | }
  (junction 92) -> (junction 178) [order 1] : [SecRwLtStLgrstUpwdStgDone]
  (junction 92) -> (junction 182) [order 2] : {SecRwLtStLgrstUpwdEn=1;}
  (junction 178) -> (junction 179)
  (junction 179) -> (junction 182)
  (junction 182) -> (junction 185)
  (junction 185) -> (junction 189) [order 1] : [SecRwLtStLgrstOtwdInwdStgDone]
  (junction 189) -> (junction 190)
  (junction 185) -> (junction 187) [order 2] : {SecRwLtStLgrstOtwdInwdEn=1;}
  (junction 190) -> (junction 187)
  (junction 187) -> (junction 10)
  (junction 10) -> (junction 12) [order 1] : [!stage1Done||(PassStFwdBkwdStgDone&&SwIntPasRecliner==0) ]
  (junction 10) -> (junction 18) [order 2] : {PassStFwdBkwdEn = 1;}
  (junction 12) -> (junction 16)
  (junction 16) -> (junction 18)
  (junction 18) -> (junction 66)
  (junction 66) -> (junction 68) [order 1] : [!stage1Done||PassStBkReclnStgDone ||(!PassStFwdBkwdStgDone && PassStBkReclnUpwdDnwdPos<=(Md30PassStBkReclnTrgtPos1))]
  (junction 66) -> (junction 72) [order 2] : {PassStBkReclnEn = 1;}
  (junction 68) -> (junction 70)
  (junction 70) -> (junction 72)
  (junction 72) -> (junction 75)
  (junction 75) -> (junction 77) [order 1] : [stage1Done&&PassStFwdBkwdStgDone &&PassStFwdBkwdPos<(PassStFwdBkwdTrgtPos1-KeSMSuFirstRwStFwdBkwdPosDelta)&&((PassStFldUpwdDnwdPos >PassStCshnFldTrgtPos1)||PassStBkReclnUpwdDnwdPos>120)]
  (junction 75) -> (junction 82) [order 2]
  (junction 77) -> (junction 80) : {FwdBkwdFailflg =1;}
  (junction 80) -> (junction 82)
  (junction 82) -> (junction 24)
  (junction 24) -> (junction 31) [order 1] : [(PassStFwdBkwdPos>=(PassStFwdBkwdTrgtPos1-KeSMSuFirstRwStFwdBkwdPosDelta))&&...
      | stage1Done]
  (junction 31) -> (junction 33) [order 1] : [PassStCshnFldStgDone ]
  (junction 33) -> (junction 56) [order 1] : [PassStFldUpwdDnwdPos >PassStCshnFldTrgtPos1]
  (junction 24) -> (junction 52) [order 2]
  (junction 31) -> (junction 35) [order 2] : {PassStCshnFldEn = 1;}
  (junction 33) -> (junction 40) [order 2]
  (junction 56) -> (junction 58) : {
      | CshnFldFailflg = 1;
      | }
  (junction 35) -> (junction 52)
  (junction 40) -> (junction 35)
  (junction 58) -> (junction 40)
  (junction 52) -> (junction 195)
  (junction 195) -> (junction 197) [order 1] : [stage2Done]
  (junction 195) -> (junction 199) [order 2]
  (junction 197) -> (junction 200) : {SecRwLtStLgrstUpwdEn=1;}
  (junction 200) -> (junction 199)
  (junction 199) -> (junction 204)
  (junction 204) -> (junction 206) [order 1] : [stage2Done]
  (junction 204) -> (junction 209) [order 2]
  (junction 206) -> (junction 208) : {SecRwLtStLgrstOtwdInwdEn=1;}
  (junction 208) -> (junction 209)
  (junction 209) -> (junction 213)
  data: stage1Done input; SecRwLtStLgrstUpwdStgDone input; SecRwLtStLgrstOtwdInwdStgDone input; SecRwLtStFtrstStgDone input; PassStBkReclnStgDone input; PassStCshnFldStgDone input; PassStFwdBkwdStgDone input; PassStFwdBkwdTrgtPos1 input; PassStCshnFldTrgtPos1 input; PassStFldUpwdDnwdPos input; PassStFwdBkwdPos input; PassStBkReclnUpwdDnwdPos input; PassStBkReclnEn output boolean; PassStCshnFldEn output boolean; PassStFwdBkwdEn output boolean; FwdBkwdFailflg output boolean; CshnFldFailflg output boolean; KeSMSuFirstRwStFwdBkwdPosDelta input; Md30PassStBkReclnTrgtPos1 input; stage2Done input; LgrstOtWdInwdPosInit input; LgrstUpDnPosinit input; LgrstOtWdInwdPos input; LgrstUpDnPos input; LgrstUpwdDnwdOpenPos1 input; SecRwLtStLgrstUpwdEn output boolean; SecRwLtStLgrstOtwdInwdEn output boolean; LgrstUpwdfailflg output boolean; stage2LgrstUpwdStgDone output boolean; stage2LgrstOtwdInwdStgDone output boolean; LgrstUpDnPosfail output boolean; LgrstOtWdInwdPosfail output boolean; SwIntPasRecliner input
  events: TrigLgrstcls output FUNCTION_CALL_EVENT
